simulink model "GNC_diagram"  (Simulink 7.1)
settings: Solver=ode45  StartTime=0.0  StopTime=10.0  RelTol=1e-3
undefined symbols (not defined in the file or in its folder): bottom_signature, sea_bottom
libraries: fordypningsprosjekt x3
settings Model: Creator=anderga  LastModifiedBy=anderga

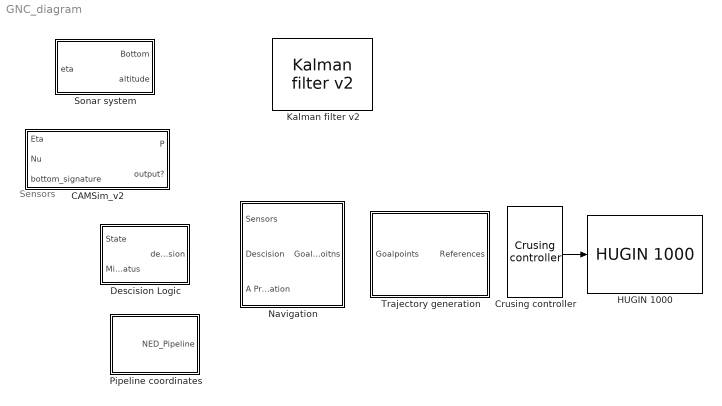
== system GNC_diagram ==
  note: Sensors
  CAMSim_v2 : Subsystem  AncestorBlock=fordypningsprosjekt/CAMSim_v2  mask{noise=on, variance=0.1}
      mask prompts: noise "Noise On?"; variance "Noise Variance"
  Crusing controller : fordypningsprosjekt/Crusing controller  SystemSampleTime=-1  Kp_u=10  Ki_u=3  Kp_c=100  Kd_c=50  Kp_d=50  Kp2_d=20  Kd_d=20
  Descision Logic : Subsystem
  HUGIN 1000 : fordypningsprosjekt/HUGIN 1000  SystemSampleTime=-1  eta_0=[0 0 0 0 0 0]  nu_0=[0 0 0 0 0 0]  c_on_off=off  beta_c=-45  V_c=0.3
  Kalman filter v2 : fordypningsprosjekt/Kalman filter v2  SystemSampleTime=-1
  Navigation : Subsystem
  Pipeline coordinates : Subsystem
  Sonar system : Subsystem  mask{sea_botto=50}
      mask prompts: sea_botto "Seabottom [m]"
      mask init:
      | load('bottom_signature')
  Trajectory generation : Subsystem
  wires:
  Crusing controller/1 -> HUGIN 1000/1

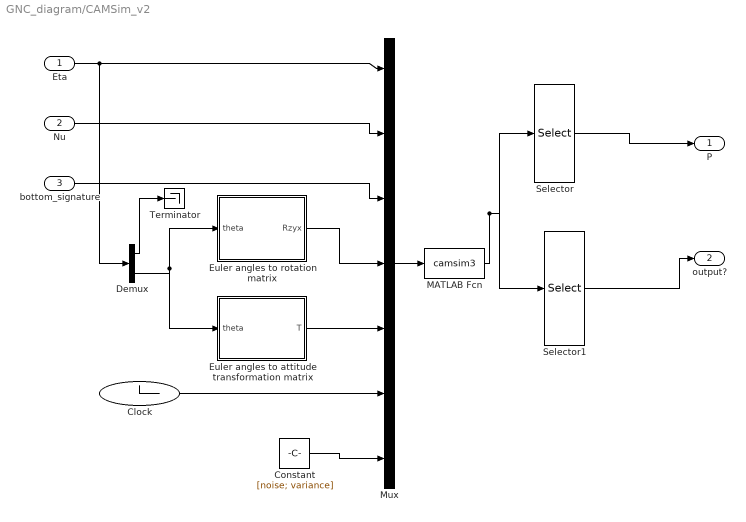
== system GNC_diagram/CAMSim_v2 ==
  Eta : Inport  OutDataType=sfix(16)  OutScaling=2^0
  Nu : Inport  Port=2  OutDataType=sfix(16)  OutScaling=2^0
  bottom_signature : Inport  Port=3  OutDataType=sfix(16)  OutScaling=2^0
  Clock : Clock
  Constant : Constant  Value=[noise; variance]  OutDataType=sfix(16)  OutScaling=2^0
  Demux : Demux  Outputs=2
  Euler angles to rotation matrix : Subsystem  AncestorBlock=marine_gnc/Models/ Kinematics/Euler angles to rotation matrix
      mask Type: Euler2R
      mask Description:
      | Determine the 3-by-3 rotation matrix from the Euler angles (roll, pitch, yaw) using the zyx convention.
      | 
      | Output is a 9x1 vector
      mask Display:
      | port_label('input',1,'theta')
      | port_label('output',1,'R')
  Euler angles to attitude transformation matrix : Subsystem  AncestorBlock=marine_gnc/Models/ Kinematics/Euler angles to attitude transformation matrix
      mask Type: Euler2T
      mask Description: Determine the 3-by-3 attitude transformation matrix  from the Euler angles (roll, pitch, yaw).
      mask Display:
      | port_label('input',1,'theta')
      | port_label('output',1,'T')
  MATLAB Fcn : MATLABFcn  MATLABFcn=camsim3  OutputDimensions=7
  Mux : Mux  Inputs=7
  Selector : Selector  InputPortWidth=7  IndexOptions=Index vector (dialog)  Indices=[1 2 3 4 5 6]  OutputSizes=1
  Selector1 : Selector  InputPortWidth=7  IndexOptions=Index vector (dialog)  Indices=[7]  OutputSizes=1
  Terminator : Terminator
  P : Outport  OutDataType=sfix(16)  OutScaling=2^0
  output? : Outport  Port=2  OutDataType=sfix(16)  OutScaling=2^0
  wires:
  Eta/1 -> Mux/1, Demux/1
  Nu/1 -> Mux/2
  bottom_signature/1 -> Mux/3
  Mux/1 -> MATLAB Fcn/1
  Demux/2 -> Euler angles to attitude transformation matrix/1(theta), Euler angles to rotation matrix/1(theta)
  Demux/1 -> Terminator/1
  Euler angles to rotation matrix/1(Rzyx) -> Mux/4
  Euler angles to attitude transformation matrix/1(T) -> Mux/5
  Clock/1 -> Mux/6
  MATLAB Fcn/1 -> Selector1/1, Selector/1
  Selector/1 -> P/1
  Selector1/1 -> output?/1
  Constant/1 -> Mux/7

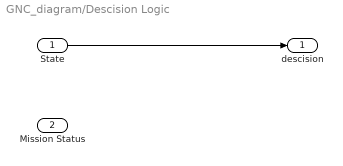
== system GNC_diagram/Descision Logic ==
  State : Inport  OutDataType=sfix(16)  OutScaling=2^0
  Mission Status : Inport  Port=2  OutDataType=sfix(16)  OutScaling=2^0
  descision : Outport  OutDataType=sfix(16)  OutScaling=2^0
  wires:
  State/1 -> descision/1

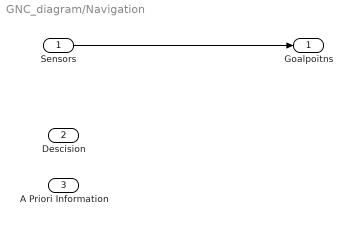
== system GNC_diagram/Navigation ==
  Sensors : Inport  OutDataType=sfix(16)  OutScaling=2^0
  Descision : Inport  Port=2  OutDataType=sfix(16)  OutScaling=2^0
  A Priori Information : Inport  Port=3  OutDataType=sfix(16)  OutScaling=2^0
  Goalpoitns : Outport  OutDataType=sfix(16)  OutScaling=2^0
  wires:
  Sensors/1 -> Goalpoitns/1

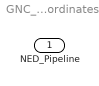
== system GNC_diagram/Pipeline coordinates ==
  NED_Pipeline : Outport  OutDataType=sfix(16)  OutScaling=2^0

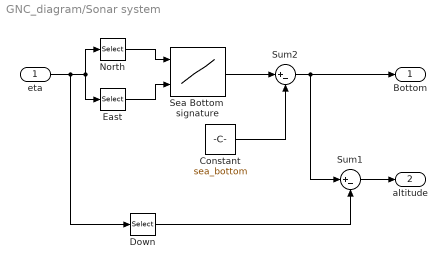
== system GNC_diagram/Sonar system ==
  eta : Inport  OutDataType=sfix(16)  OutScaling=2^0
  Constant : Constant  Value=sea_bottom  OutDataType=sfix(16)  OutScaling=2^0
  Down : Selector  InputPortWidth=6  IndexOptions=Index vector (dialog)  Indices=[3]  OutputSizes=1
  East : Selector  InputPortWidth=6  IndexOptions=Index vector (dialog)  Indices=[2]  OutputSizes=1
  North : Selector  InputPortWidth=6  IndexOptions=Index vector (dialog)  Indices=[1]  OutputSizes=1
  Sea Bottom  signature : Lookup2D  RowIndex=[1:size(bottom_signature)]  ColumnIndex=[1:size(bottom_signature)]  Table=bottom_signature  LookUpMeth=Use Input Nearest  OutDataType=sfix(16)  OutScaling=2^0
  Sum1 : Sum  Inputs=|+-  OutDataType=sfix(16)  OutScaling=2^0
  Sum2 : Sum  Inputs=|+-  OutDataType=sfix(16)  OutScaling=2^0
  Bottom : Outport  OutDataType=sfix(16)  OutScaling=2^0
  altitude : Outport  Port=2  OutDataType=sfix(16)  OutScaling=2^0
  wires:
  Down/1 -> Sum1/2
  Sum1/1 -> altitude/1
  North/1 -> Sea Bottom  signature/1
  eta/1 -> North/1, East/1, Down/1
  East/1 -> Sea Bottom  signature/2
  Sea Bottom  signature/1 -> Sum2/1
  Sum2/1 -> Sum1/1, Bottom/1
  Constant/1 -> Sum2/2

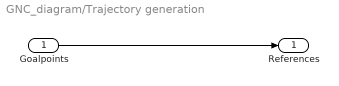
== system GNC_diagram/Trajectory generation ==
  Goalpoints : Inport  OutDataType=sfix(16)  OutScaling=2^0
  References : Outport  OutDataType=sfix(16)  OutScaling=2^0
  wires:
  Goalpoints/1 -> References/1

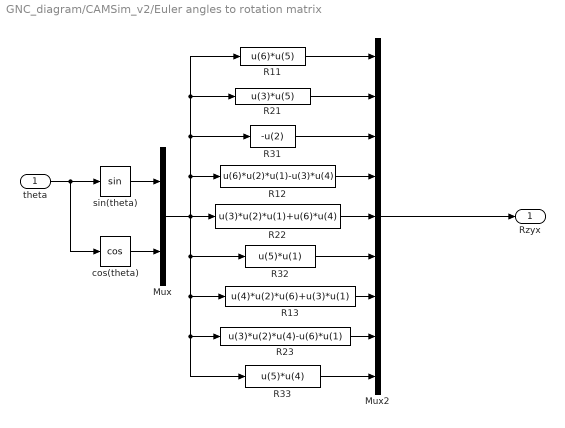
== system GNC_diagram/CAMSim_v2/Euler angles to rotation matrix ==
  theta : Inport  OutDataType=sfix(16)  OutScaling=2^0
  Mux : Mux  Inputs=2
  Mux2 : Mux  Inputs=9
  R11 : Fcn  Expr=u(6)*u(5)
  R12 : Fcn  Expr=u(6)*u(2)*u(1)-u(3)*u(4)
  R13 : Fcn  Expr=u(4)*u(2)*u(6)+u(3)*u(1)
  "R21 " : Fcn  Expr=u(3)*u(5)
  R22 : Fcn  Expr=u(3)*u(2)*u(1)+u(6)*u(4)
  R23 : Fcn  Expr=u(3)*u(2)*u(4)-u(6)*u(1)
  "R31 " : Fcn  Expr=-u(2)
  R32 : Fcn  Expr=u(5)*u(1)
  R33 : Fcn  Expr=u(5)*u(4)
  cos(theta) : Trigonometry  Operator=cos
  sin(theta) : Trigonometry
  Rzyx : Outport  OutDataType=sfix(16)  OutScaling=2^0  InitialOutput=0
  wires:
  R33/1 -> Mux2/9
  R32/1 -> Mux2/6
  "R21 "/1 -> Mux2/2
  "R31 "/1 -> Mux2/3
  R12/1 -> Mux2/4
  R22/1 -> Mux2/5
  R13/1 -> Mux2/7
  R23/1 -> Mux2/8
  Mux/1 -> R12/1, "R21 "/1, R11/1, "R31 "/1, R22/1, R23/1, R33/1, R13/1, R32/1
  theta/1 -> cos(theta)/1, sin(theta)/1
  cos(theta)/1 -> Mux/2
  sin(theta)/1 -> Mux/1
  Mux2/1 -> Rzyx/1
  R11/1 -> Mux2/1

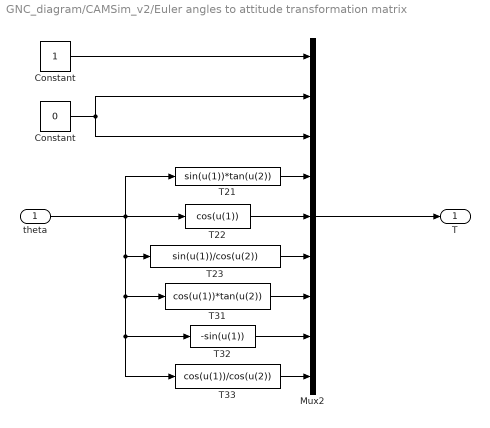
== system GNC_diagram/CAMSim_v2/Euler angles to attitude transformation matrix ==
  theta : Inport  OutDataType=sfix(16)  OutScaling=2^0
  Constant : Constant  OutDataType=sfix(16)  OutScaling=2^0
  "Constant " : Constant  Value=0  OutDataType=sfix(16)  OutScaling=2^0
  Mux2 : Mux  Inputs=9
  "T21 " : Fcn  Expr=sin(u(1))*tan(u(2))
  T22 : Fcn  Expr=cos(u(1))
  T23 : Fcn  Expr=sin(u(1))/cos(u(2))
  "T31 " : Fcn  Expr=cos(u(1))*tan(u(2))
  T32 : Fcn  Expr=-sin(u(1))
  T33 : Fcn  Expr=cos(u(1))/cos(u(2))
  T : Outport  OutDataType=sfix(16)  OutScaling=2^0  InitialOutput=0
  wires:
  T32/1 -> Mux2/8
  "T31 "/1 -> Mux2/7
  "T21 "/1 -> Mux2/4
  "Constant "/1 -> Mux2/3, Mux2/2
  T33/1 -> Mux2/9
  T22/1 -> Mux2/5
  T23/1 -> Mux2/6
  theta/1 -> "T21 "/1, T22/1, "T31 "/1, T32/1, T33/1, T23/1
  Mux2/1 -> T/1
  Constant/1 -> Mux2/1
